simulink model "linear_validation"  (R2017b)
settings: Solver=VariableStepAuto  StartTime=0.0  StopTime=10.0  RelTol=1e-3
undefined symbols (not defined in the file): system
settings Model: Creator=Twan  LastModifiedBy=Raffi

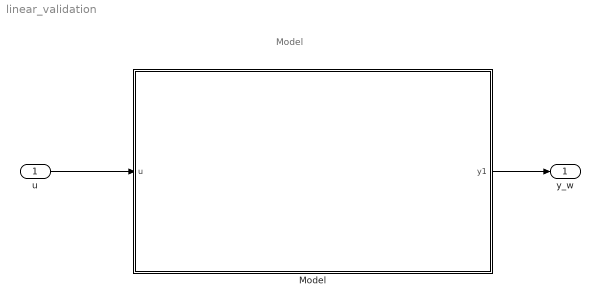
== system linear_validation ==
  note: Model
  u : Inport
  Model : Subsystem
  "y_w " : Outport
  wires:
  Model/1(y1) -> "y_w "/1
  u/1 -> Model/1(u)

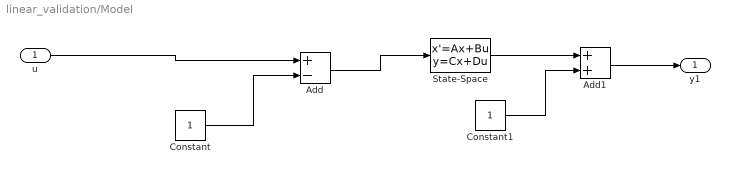
== system linear_validation/Model ==
  u : Inport
  Add : Sum  Inputs=+-
  Add1 : Sum
  Constant : Constant
  Constant1 : Constant
  State-Space : StateSpace  A=system.ss.lin.A  B=system.ss.lin.B  C=system.ss.lin.C  D=system.ss.lin.D  InitialCondition=[0]
  y1 : Outport
  wires:
  u/1 -> Add/1
  Constant/1 -> Add/2
  Add/1 -> State-Space/1
  State-Space/1 -> Add1/1
  Constant1/1 -> Add1/2
  Add1/1 -> y1/1
